simulink model "kalman_onefile"  (R2013b)
settings: Solver=ode3  StartTime=100  StopTime=200  FixedStep=0.1  RelTol=1e-3
settings Model: Creator=Franta  LastModifiedBy=Franta

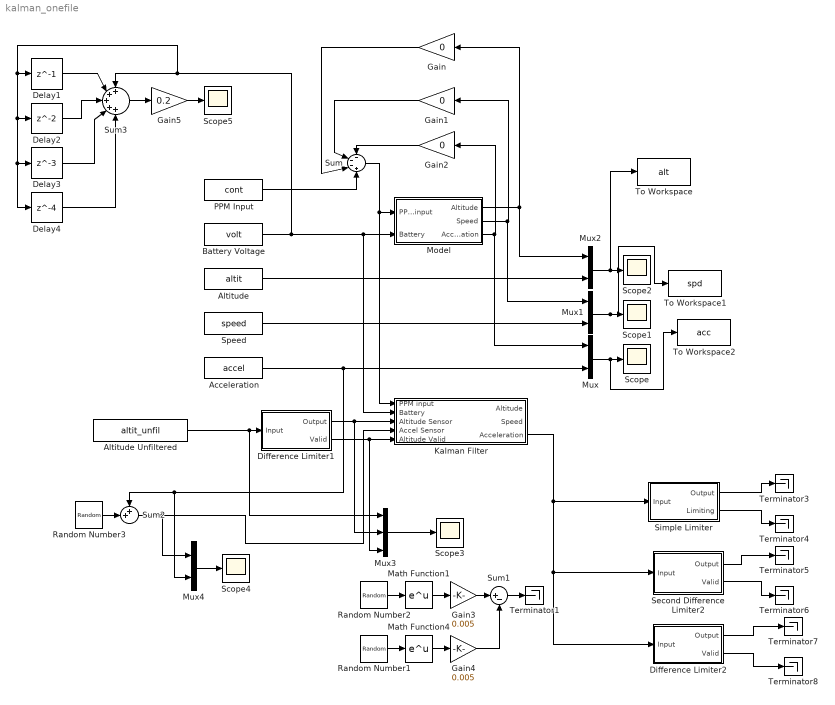
== system kalman_onefile ==
  Acceleration : FromWorkspace  VariableName=accel  SampleTime=0  OutputAfterFinalValue=Holding final value
  Altitude : FromWorkspace  VariableName=altit  SampleTime=0  OutputAfterFinalValue=Holding final value
  Altitude Unfiltered : FromWorkspace  VariableName=altit_unfil  SampleTime=0  OutputAfterFinalValue=Holding final value
  Battery Voltage : FromWorkspace  VariableName=volt  SampleTime=0  OutputAfterFinalValue=Holding final value
  Delay1 : Delay  DelayLength=1  InitialCondition=11
  Delay2 : Delay  InitialCondition=11
  Delay3 : Delay  DelayLength=3  InitialCondition=11
  Delay4 : Delay  DelayLength=4  InitialCondition=11
  Difference Limiter1 : Subsystem
  Difference Limiter2 : Subsystem
  Gain : Gain  Gain=0
  Gain1 : Gain  Gain=0
  Gain2 : Gain  Gain=0
  Gain3 : Gain  Gain=0.005
  Gain4 : Gain  Gain=0.005
  Gain5 : Gain  Gain=0.2
  Kalman Filter : Subsystem
  Math Function1 : Math  SaturateOnIntegerOverflow=on
  Math Function4 : Math  SaturateOnIntegerOverflow=on
  Model : Subsystem
  Mux{,1..2,4} (4 alike) : Mux  Inputs=2
  Mux3 : Mux  Inputs=3
  PPM Input : FromWorkspace  VariableName=cont  SampleTime=0  OutputAfterFinalValue=Holding final value
  Random Number1 : RandomNumber  Variance=4  Seed=1  SampleTime=0.1
  Random Number2 : RandomNumber  Variance=4  SampleTime=0.1
  Random Number3 : RandomNumber  Variance=0.1  SampleTime=0.1
  Scope{,1..5} (6 alike) : Scope
      Scope settings: YMin=0  YMax=47.5
      Scope1 settings: TimeRange=50
      Scope2 settings: SaveName=ScopeData2
      Scope3 settings: YMin=0  YMax=47.5  SaveName=ScopeData3
      Scope4 settings: YMin=0  YMax=47.5  SaveName=ScopeData4
      Scope5 settings: SaveName=ScopeData5
  Second Difference Limiter2 : Subsystem
  Simple Limiter : Subsystem
  Speed : FromWorkspace  VariableName=speed  SampleTime=0  OutputAfterFinalValue=Holding final value
  Sum : Sum  Inputs=---+
  Sum1 : Sum  Inputs=|+-
  Sum2 : Sum  Inputs=++|
  Sum3 : Sum  Inputs=+++++
  Terminator{1,3..8} (7 alike) : Terminator
  To Workspace : ToWorkspace  VariableName=alt  SampleTime=-1  SaveFormat=Timeseries
  To Workspace1 : ToWorkspace  VariableName=spd  SampleTime=-1  SaveFormat=Timeseries
  To Workspace2 : ToWorkspace  VariableName=acc  SampleTime=-1  SaveFormat=Timeseries
  wires:
  Kalman Filter/3(Acceleration) -> Difference Limiter2/1(Input), Second Difference Limiter2/1(Input), Simple Limiter/1(Input)
  Simple Limiter/1(Output) -> Terminator3/1
  Simple Limiter/2(Limiting) -> Terminator4/1
  Mux3/1 -> Scope3/1
  Second Difference Limiter2/1(Output) -> Terminator5/1
  Second Difference Limiter2/2(Valid) -> Terminator6/1
  Model/1(Altitude) -> Gain/1, Mux2/1
  Model/2(Speed) -> Mux1/1, Gain1/1
  Model/3(Acceleration) -> Mux/1, Gain2/1
  Sum/1 -> Kalman Filter/1(PPM input), Model/1(PPM input)
  Gain2/1 -> Sum/1
  Gain1/1 -> Sum/2
  Gain/1 -> Sum/3
  PPM Input/1 -> Sum/4
  Difference Limiter2/1(Output) -> Terminator7/1
  Difference Limiter2/2(Valid) -> Terminator8/1
  Difference Limiter1/1(Output) -> Kalman Filter/3(Altitude Sensor), Mux3/2
  Difference Limiter1/2(Valid) -> Mux3/3, Kalman Filter/5(Altitude Valid)
  Speed/1 -> Mux1/2
  Random Number2/1 -> Math Function1/1
  Math Function1/1 -> Gain3/1
  Random Number1/1 -> Math Function4/1
  Math Function4/1 -> Gain4/1
  Gain4/1 -> Sum1/2
  Gain3/1 -> Sum1/1
  Altitude Unfiltered/1 -> Mux3/1, Difference Limiter1/1(Input)
  Sum1/1 -> Terminator1/1
  Altitude/1 -> Mux2/2
  Random Number3/1 -> Sum2/2
  Sum2/1 -> Mux4/1, Kalman Filter/4(Accel Sensor)
  Mux4/1 -> Scope4/1
  Acceleration/1 -> Mux4/2, Sum2/1, Mux/2
  Mux/1 -> To Workspace2/1, Scope/1
  Mux1/1 -> To Workspace1/1, Scope1/1
  Mux2/1 -> To Workspace/1, Scope2/1
  Battery Voltage/1 -> Delay4/1, Delay3/1, Delay2/1, Delay1/1, Sum3/1, Kalman Filter/2(Battery), Model/2(Battery)
  Delay1/1 -> Sum3/2
  Delay2/1 -> Sum3/3
  Delay3/1 -> Sum3/4
  Delay4/1 -> Sum3/5
  Sum3/1 -> Gain5/1
  Gain5/1 -> Scope5/1

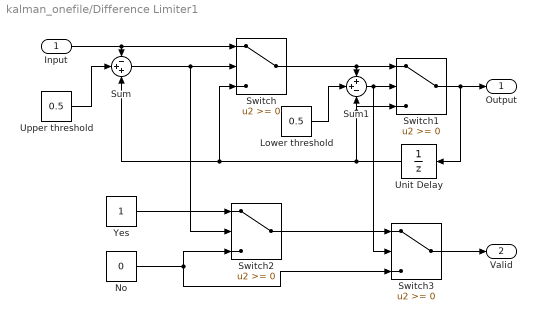
== system kalman_onefile/Difference Limiter1 ==
  Input : Inport
  Lower threshold : Constant  Value=0.5
  No : Constant  Value=0
  Sum : Sum  Inputs=-++
  Sum1 : Sum  Inputs=++-
  Switch{,1..3} (4 alike) : Switch
  Unit Delay : UnitDelay  InitialCondition=1  SampleTime=-1
  Upper threshold : Constant  Value=0.5
  Yes : Constant
  Output : Outport
  Valid : Outport  Port=2
  wires:
  Switch3/1 -> Valid/1
  Switch2/1 -> Switch3/1
  No/1 -> Switch3/3, Switch2/3
  Yes/1 -> Switch2/1
  Sum1/1 -> Switch1/2, Switch3/2
  Sum/1 -> Switch/2, Switch2/2
  Unit Delay/1 -> Sum1/3, Switch1/3, Switch/3, Sum/3
  Input/1 -> Sum/1, Switch/1
  Upper threshold/1 -> Sum/2
  Switch1/1 -> Output/1, Unit Delay/1
  Switch/1 -> Sum1/1, Switch1/1
  Lower threshold/1 -> Sum1/2

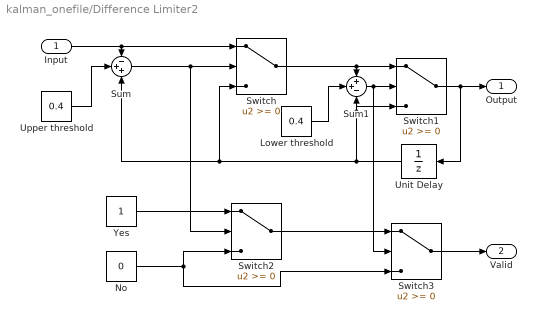
== system kalman_onefile/Difference Limiter2 ==
  Input : Inport
  Lower threshold : Constant  Value=0.4
  No : Constant  Value=0
  Sum : Sum  Inputs=-++
  Sum1 : Sum  Inputs=++-
  Switch{,1..3} (4 alike) : Switch
  Unit Delay : UnitDelay  InitialCondition=1  SampleTime=-1
  Upper threshold : Constant  Value=0.4
  Yes : Constant
  Output : Outport
  Valid : Outport  Port=2
  wires:
  Lower threshold/1 -> Sum1/2
  Switch/1 -> Switch1/1, Sum1/1
  Switch1/1 -> Unit Delay/1, Output/1
  Upper threshold/1 -> Sum/2
  Input/1 -> Switch/1, Sum/1
  Unit Delay/1 -> Sum/3, Switch/3, Switch1/3, Sum1/3
  Sum/1 -> Switch2/2, Switch/2
  Sum1/1 -> Switch3/2, Switch1/2
  Yes/1 -> Switch2/1
  No/1 -> Switch2/3, Switch3/3
  Switch2/1 -> Switch3/1
  Switch3/1 -> Valid/1

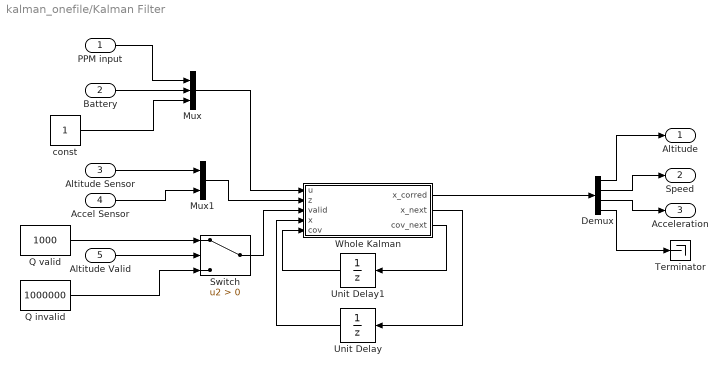
== system kalman_onefile/Kalman Filter ==
  PPM input : Inport
  Battery : Inport  Port=2
  Altitude Sensor : Inport  Port=3
  Accel Sensor : Inport  Port=4
  Altitude Valid : Inport  Port=5
  Demux : Demux
  Mux : Mux  Inputs=3
  Mux1 : Mux  Inputs=2
  Q invalid : Constant  Value=1000000
  Q valid : Constant  Value=1000
  Switch : Switch  Criteria=u2 > Threshold
  Terminator : Terminator
  Unit Delay : UnitDelay  InitialCondition=[0 0 0 0]'  SampleTime=-1
  Unit Delay1 : UnitDelay  InitialCondition=[1 0 0 0; 0 1 0 0; 0 0 1 0; 0 0 0 1]  SampleTime=-1
  Whole Kalman : MATLAB Function  TreatAsAtomicUnit=on
  const : Constant
  Altitude : Outport
  Speed : Outport  Port=2
  Acceleration : Outport  Port=3
  wires:
  Whole Kalman/1(x_corred) -> Demux/1
  Mux/1 -> Whole Kalman/1(u)
  PPM input/1 -> Mux/1
  Battery/1 -> Mux/2
  const/1 -> Mux/3
  Demux/2 -> Speed/1
  Demux/3 -> Acceleration/1
  Demux/1 -> Altitude/1
  Demux/4 -> Terminator/1
  Unit Delay1/1 -> Whole Kalman/5(cov)
  Whole Kalman/3(cov_next) -> Unit Delay1/1
  Whole Kalman/2(x_next) -> Unit Delay/1
  Unit Delay/1 -> Whole Kalman/4(x)
  Q valid/1 -> Switch/1
  Switch/1 -> Whole Kalman/3(valid)
  Q invalid/1 -> Switch/3
  Altitude Valid/1 -> Switch/2
  Altitude Sensor/1 -> Mux1/1
  Accel Sensor/1 -> Mux1/2
  Mux1/1 -> Whole Kalman/2(z)

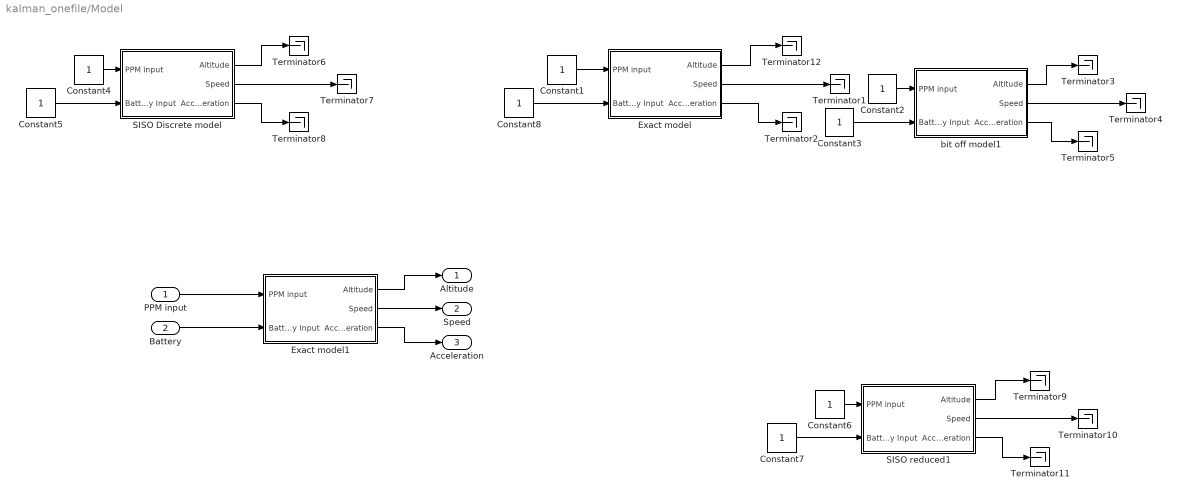
== system kalman_onefile/Model ==
  PPM input : Inport
  Battery : Inport  Port=2
  Constant{1..8} (8 alike) : Constant
  Exact model : Subsystem
  Exact model1 : Subsystem
  SISO Discrete model : Subsystem
  SISO reduced1 : Subsystem
  Terminator{1..12} (12 alike) : Terminator
  bit off model1 : Subsystem
  Altitude : Outport
  Speed : Outport  Port=2
  Acceleration : Outport  Port=3
  wires:
  bit off model1/1(Altitude) -> Terminator3/1
  bit off model1/2(Speed) -> Terminator4/1
  bit off model1/3(Acceleration) -> Terminator5/1
  Constant3/1 -> bit off model1/2(Battery Input)
  Constant2/1 -> bit off model1/1(PPM input)
  SISO Discrete model/1(Altitude) -> Terminator6/1
  SISO Discrete model/2(Speed) -> Terminator7/1
  SISO Discrete model/3(Acceleration) -> Terminator8/1
  Constant5/1 -> SISO Discrete model/2(Battery Input)
  Constant4/1 -> SISO Discrete model/1(PPM input)
  PPM input/1 -> Exact model1/1(PPM input)
  Constant8/1 -> Exact model/2(Battery Input)
  Constant1/1 -> Exact model/1(PPM input)
  Exact model/1(Altitude) -> Terminator12/1
  Exact model/2(Speed) -> Terminator1/1
  Exact model/3(Acceleration) -> Terminator2/1
  Battery/1 -> Exact model1/2(Battery Input)
  Exact model1/1(Altitude) -> Altitude/1
  Exact model1/2(Speed) -> Speed/1
  Exact model1/3(Acceleration) -> Acceleration/1
  SISO reduced1/1(Altitude) -> Terminator9/1
  SISO reduced1/2(Speed) -> Terminator10/1
  SISO reduced1/3(Acceleration) -> Terminator11/1
  Constant7/1 -> SISO reduced1/2(Battery Input)
  Constant6/1 -> SISO reduced1/1(PPM input)

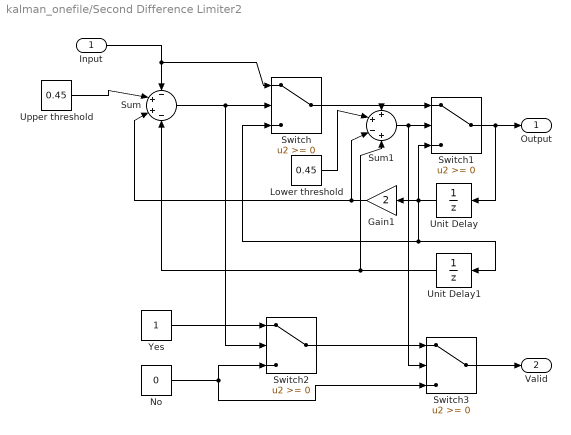
== system kalman_onefile/Second Difference Limiter2 ==
  Input : Inport
  Gain1 : Gain  Gain=2
  Lower threshold : Constant  Value=0.45
  No : Constant  Value=0
  Sum : Sum  Inputs=-++-
  Sum1 : Sum  Inputs=++-+
  Switch{,1..3} (4 alike) : Switch
  Unit Delay : UnitDelay  InitialCondition=1  SampleTime=-1
  Unit Delay1 : UnitDelay  InitialCondition=1  SampleTime=-1
  Upper threshold : Constant  Value=0.45
  Yes : Constant
  Output : Outport
  Valid : Outport  Port=2
  wires:
  Gain1/1 -> Sum1/3, Sum/3
  Switch3/1 -> Valid/1
  Switch2/1 -> Switch3/1
  No/1 -> Switch3/3, Switch2/3
  Yes/1 -> Switch2/1
  Sum1/1 -> Switch1/2, Switch3/2
  Sum/1 -> Switch2/2, Switch/2
  Unit Delay/1 -> Gain1/1, Switch1/3, Unit Delay1/1, Switch/3
  Input/1 -> Switch/1, Sum/1
  Upper threshold/1 -> Sum/2
  Switch1/1 -> Output/1, Unit Delay/1
  Switch/1 -> Switch1/1, Sum1/1
  Lower threshold/1 -> Sum1/2
  Unit Delay1/1 -> Sum1/4, Sum/4

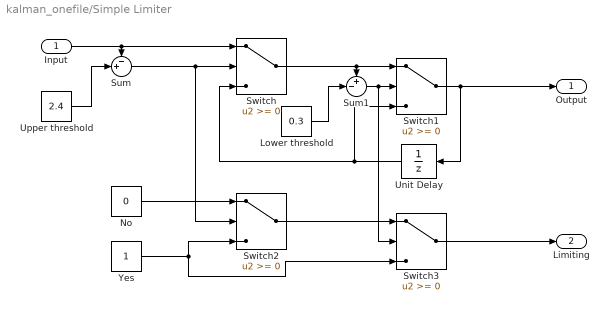
== system kalman_onefile/Simple Limiter ==
  Input : Inport
  Lower threshold : Constant  Value=0.3
  No : Constant  Value=0
  Sum : Sum  Inputs=-+|
  Sum1 : Sum  Inputs=+-|
  Switch{,1..3} (4 alike) : Switch
  Unit Delay : UnitDelay  SampleTime=-1
  Upper threshold : Constant  Value=2.4
  Yes : Constant
  Output : Outport
  Limiting : Outport  Port=2
  wires:
  Unit Delay/1 -> Switch1/3, Switch/3
  Sum/1 -> Switch2/2, Switch/2
  Input/1 -> Sum/1, Switch/1
  Upper threshold/1 -> Sum/2
  Switch1/1 -> Output/1, Unit Delay/1
  Sum1/1 -> Switch3/2, Switch1/2
  Switch/1 -> Sum1/1, Switch1/1
  Lower threshold/1 -> Sum1/2
  No/1 -> Switch2/1
  Yes/1 -> Switch2/3, Switch3/3
  Switch2/1 -> Switch3/1
  Switch3/1 -> Limiting/1

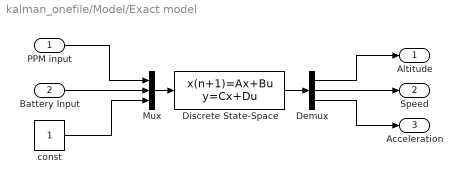
== system kalman_onefile/Model/Exact model ==
  PPM input : Inport
  Battery Input : Inport  Port=2
  Demux : Demux  Outputs=3
  Discrete State-Space : DiscreteStateSpace  A=[1 0.1 0 0; 0 1 0.1 0; 0 0 0 1; 0 0 -0.6466 1.5736]  B=[0 0 0; 0 0 0; 0.002711 0.003372 -17.7363; 0.001897 0.08581 -13.3891]  C=[1 0 0 0; 0 1 0 0; 0 0 1 0]  D=[0 0 0; 0 0 0; 0 0 0]  SampleTime=0.1
  Mux : Mux  Inputs=3
  const : Constant
  Altitude : Outport
  Speed : Outport  Port=2
  Acceleration : Outport  Port=3
  wires:
  const/1 -> Mux/3
  Battery Input/1 -> Mux/2
  PPM input/1 -> Mux/1
  Discrete State-Space/1 -> Demux/1
  Demux/3 -> Acceleration/1
  Demux/2 -> Speed/1
  Demux/1 -> Altitude/1
  Mux/1 -> Discrete State-Space/1

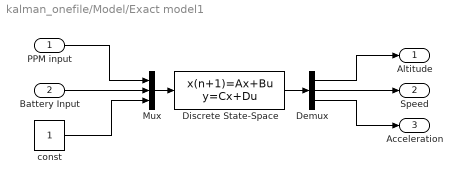
== system kalman_onefile/Model/Exact model1 ==
  PPM input : Inport
  Battery Input : Inport  Port=2
  Demux : Demux  Outputs=3
  Discrete State-Space : DiscreteStateSpace  A=[1 0.1 0 0; 0 1 0.1 0; 0 0 0 1; 0 0 -0.6466 1.5736]  B=[0 0 0; 0 0 0; 0.002711 0.003372 -17.7363; 0.001897 0.08581 -13.3891]  C=[1 0 0 0; 0 1 0 0; 0 0 1 0]  D=[0 0 0; 0 0 0; 0 0 0]  X0=[0 -0.5 0 0]  SampleTime=0.1
  Mux : Mux  Inputs=3
  const : Constant
  Altitude : Outport
  Speed : Outport  Port=2
  Acceleration : Outport  Port=3
  wires:
  Mux/1 -> Discrete State-Space/1
  Demux/1 -> Altitude/1
  Demux/2 -> Speed/1
  Demux/3 -> Acceleration/1
  Discrete State-Space/1 -> Demux/1
  PPM input/1 -> Mux/1
  Battery Input/1 -> Mux/2
  const/1 -> Mux/3

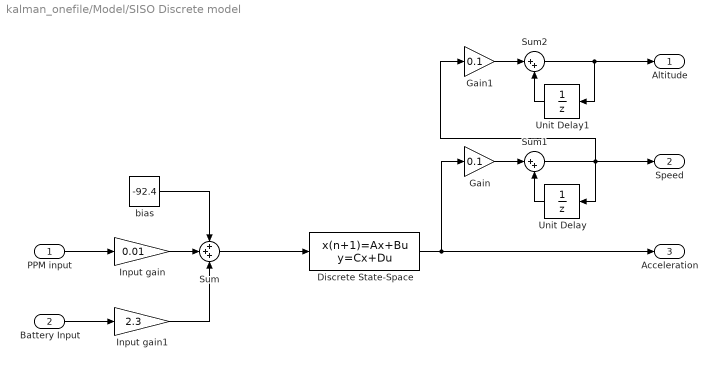
== system kalman_onefile/Model/SISO Discrete model ==
  PPM input : Inport
  Battery Input : Inport  Port=2
  Discrete State-Space : DiscreteStateSpace  A=[0 1; -0.67523 1.64069]  B=[0.28811; 0.18591]  C=[1 0]  D=0  SampleTime=0.1
  Gain : Gain  Gain=0.1
  Gain1 : Gain  Gain=0.1
  Input gain : Gain  Gain=0.01
  Input gain1 : Gain  Gain=2.3
  Sum : Sum  Inputs=+++
  Sum1 : Sum  Inputs=|++
  Sum2 : Sum  Inputs=|++
  Unit Delay : UnitDelay  SampleTime=-1
  Unit Delay1 : UnitDelay  InitialCondition=1  SampleTime=-1
  bias : Constant  Value=-92.4
  Altitude : Outport
  Speed : Outport  Port=2
  Acceleration : Outport  Port=3
  wires:
  PPM input/1 -> Input gain/1
  Battery Input/1 -> Input gain1/1
  Input gain/1 -> Sum/2
  Input gain1/1 -> Sum/3
  bias/1 -> Sum/1
  Sum/1 -> Discrete State-Space/1
  Discrete State-Space/1 -> Gain/1, Acceleration/1
  Unit Delay/1 -> Sum1/2
  Sum1/1 -> Unit Delay/1, Gain1/1, Speed/1
  Sum2/1 -> Unit Delay1/1, Altitude/1
  Unit Delay1/1 -> Sum2/2
  Gain/1 -> Sum1/1
  Gain1/1 -> Sum2/1

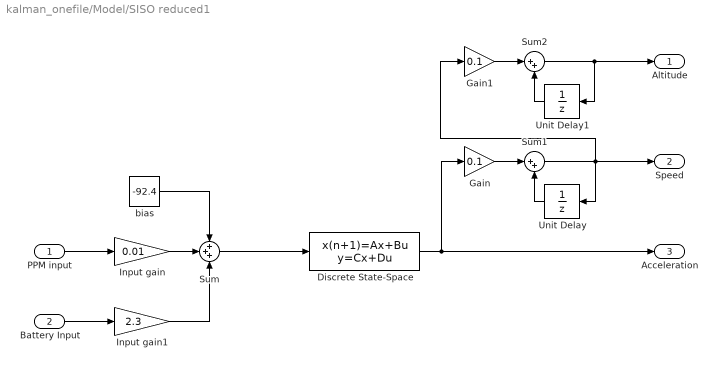
== system kalman_onefile/Model/SISO reduced1 ==
  PPM input : Inport
  Battery Input : Inport  Port=2
  Discrete State-Space : DiscreteStateSpace  A=[0.6292]  B=[0.2769]  C=[1]  D=0  SampleTime=0.1
  Gain : Gain  Gain=0.1
  Gain1 : Gain  Gain=0.1
  Input gain : Gain  Gain=0.01
  Input gain1 : Gain  Gain=2.3
  Sum : Sum  Inputs=+++
  Sum1 : Sum  Inputs=|++
  Sum2 : Sum  Inputs=|++
  Unit Delay : UnitDelay  SampleTime=-1
  Unit Delay1 : UnitDelay  InitialCondition=1  SampleTime=-1
  bias : Constant  Value=-92.4
  Altitude : Outport
  Speed : Outport  Port=2
  Acceleration : Outport  Port=3
  wires:
  PPM input/1 -> Input gain/1
  Battery Input/1 -> Input gain1/1
  Input gain/1 -> Sum/2
  Input gain1/1 -> Sum/3
  bias/1 -> Sum/1
  Sum/1 -> Discrete State-Space/1
  Discrete State-Space/1 -> Gain/1, Acceleration/1
  Unit Delay/1 -> Sum1/2
  Sum1/1 -> Unit Delay/1, Gain1/1, Speed/1
  Sum2/1 -> Unit Delay1/1, Altitude/1
  Unit Delay1/1 -> Sum2/2
  Gain/1 -> Sum1/1
  Gain1/1 -> Sum2/1

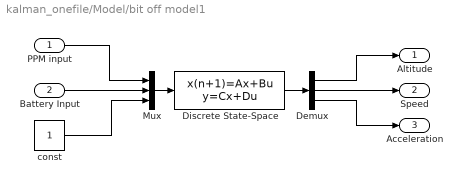
== system kalman_onefile/Model/bit off model1 ==
  PPM input : Inport
  Battery Input : Inport  Port=2
  Demux : Demux  Outputs=3
  Discrete State-Space : DiscreteStateSpace  A=[1 0.1 0 0; 0 1 0.1 0; 0 0 0 0.99; 0 0 -0.6966 1.5736]  B=[0 0 0; 0 0 0; 0.002711 0.003372 -17.7363; 0.001897 0.08581 -13.3891]  C=[1 0 0 0; 0 1 0 0; 0 0 1 0]  D=[0 0 0; 0 0 0; 0 0 0]  SampleTime=0.1
  Mux : Mux  Inputs=3
  const : Constant
  Altitude : Outport
  Speed : Outport  Port=2
  Acceleration : Outport  Port=3
  wires:
  Mux/1 -> Discrete State-Space/1
  Demux/1 -> Altitude/1
  Demux/2 -> Speed/1
  Demux/3 -> Acceleration/1
  Discrete State-Space/1 -> Demux/1
  PPM input/1 -> Mux/1
  Battery Input/1 -> Mux/2
  const/1 -> Mux/3

== matlab function kalman_onefile/Kalman Filter/Whole Kalman ==
  data: u input; z input; valid input; x_corred output; x input; cov input; x_next output; cov_next output
function [x_corred, x_next, cov_next] = kalman(u, z, valid, x, cov)
A = [1 0.1 0 0; 0 1 0.1 0; 0 0 0 1; 0 0 -0.6466 1.5736];
B = [0 0 0; 0 0 0; 0.002711 0.003372 -17.7363; 0.001897 0.08581 -13.3891];
P = [1 0 0 0; 0 0 1 0];
Q = [1000/(valid + 0.001) 0; 0 100];
R = [1 0 0 0; 0 1 0 0; 0 0 1 0; 0 0 0 1];
K = (cov*P')/((P*cov*P') + Q);
x_corred = x + K*(z - P*x);
cov_corred = (eye(4) - K*P)*cov;
x_next = A*x_corred + B*u;
cov_next = (A*cov_corred*A') + R;
end
